simulink model "ctrl_custom"  (R2016b)
settings: Solver=ode4  StartTime=0.0  StopTime=inf  FixedStep=0.01  RelTol=1e-3  EnableMultiTasking=on
values from neighbouring files (symbols this model uses):
  T_pinv = T'*inv(T*T')    [initfile.m]
libraries: marine_gnc x8, simulink x1
(part 3 of 3)

== system ctrl_custom/Observer output /b_hat output ==
  b_hat : Inport
  Demux : Demux  Outputs=3
  b_psi_hat : S-Function  Priority=3  FunctionName=NIVeriStandIO  Parameters=width dtype portnum stime stype btype  SFunctionDeploymentMode=off  EnableBusSupport=off  mask(NI VeriStand Outport){portnum=3, width=-1, stime=-1, dtype=auto, stype=auto, btype=0}
      mask prompts: portnum "Port number:"; width "Port dimensions (-1 for dynamically sized):"; stime "Sample time (-1 for inherited):"; dtype "Data type:"; stype "Signal type:"; btype "Block type:"
      mask help: Use this outport on any level of nested subsystems to allow NI VeriStand software to map signals to it.
      mask init:
      | NIVeriStandIO_init;
      settings: CopyFcn=NIVeriStand_MDL_functions('', 'IO_copy');  DeleteFcn=NIVeriStand_MDL_functions('', 'IO_delete');  MoveFcn=set_param(gcb, 'Mask', 'on');
      mask Callback portnum: NIVeriStand_MDL_functions('', 'IO_setportnum');
      mask TypeOptions dtype: auto | double | single | int8 | uint8 | int16 | uint16 | int32 | uint32 | boolean
      mask Callback dtype: NIVeriStand_MDL_functions('', 'IO_booleansignal');
      mask TypeOptions stype: auto | real | complex
      mask Display:
      | patch([-x x], [-y y], [.90980 .81960 .32156]);
      | plot([xrad -x x xrad], [yrad -y y yrad]);
      | fprintf('NI Out%d', portnum);
  b_x_hat : S-Function  Priority=1  FunctionName=NIVeriStandIO  Parameters=width dtype portnum stime stype btype  SFunctionDeploymentMode=off  EnableBusSupport=off  mask(NI VeriStand Outport){portnum=1, width=-1, stime=-1, dtype=auto, stype=auto, btype=0}
      mask prompts: portnum "Port number:"; width "Port dimensions (-1 for dynamically sized):"; stime "Sample time (-1 for inherited):"; dtype "Data type:"; stype "Signal type:"; btype "Block type:"
      mask help: Use this outport on any level of nested subsystems to allow NI VeriStand software to map signals to it.
      mask init:
      | NIVeriStandIO_init;
      settings: CopyFcn=NIVeriStand_MDL_functions('', 'IO_copy');  DeleteFcn=NIVeriStand_MDL_functions('', 'IO_delete');  MoveFcn=set_param(gcb, 'Mask', 'on');
      mask Callback portnum: NIVeriStand_MDL_functions('', 'IO_setportnum');
      mask TypeOptions dtype: auto | double | single | int8 | uint8 | int16 | uint16 | int32 | uint32 | boolean
      mask Callback dtype: NIVeriStand_MDL_functions('', 'IO_booleansignal');
      mask TypeOptions stype: auto | real | complex
      mask Display:
      | patch([-x x], [-y y], [.90980 .81960 .32156]);
      | plot([xrad -x x xrad], [yrad -y y yrad]);
      | fprintf('NI Out%d', portnum);
  b_y_hat : S-Function  Priority=2  FunctionName=NIVeriStandIO  Parameters=width dtype portnum stime stype btype  SFunctionDeploymentMode=off  EnableBusSupport=off  mask(NI VeriStand Outport){portnum=2, width=-1, stime=-1, dtype=auto, stype=auto, btype=0}
      mask prompts: portnum "Port number:"; width "Port dimensions (-1 for dynamically sized):"; stime "Sample time (-1 for inherited):"; dtype "Data type:"; stype "Signal type:"; btype "Block type:"
      mask help: Use this outport on any level of nested subsystems to allow NI VeriStand software to map signals to it.
      mask init:
      | NIVeriStandIO_init;
      settings: CopyFcn=NIVeriStand_MDL_functions('', 'IO_copy');  DeleteFcn=NIVeriStand_MDL_functions('', 'IO_delete');  MoveFcn=set_param(gcb, 'Mask', 'on');
      mask Callback portnum: NIVeriStand_MDL_functions('', 'IO_setportnum');
      mask TypeOptions dtype: auto | double | single | int8 | uint8 | int16 | uint16 | int32 | uint32 | boolean
      mask Callback dtype: NIVeriStand_MDL_functions('', 'IO_booleansignal');
      mask TypeOptions stype: auto | real | complex
      mask Display:
      | patch([-x x], [-y y], [.90980 .81960 .32156]);
      | plot([xrad -x x xrad], [yrad -y y yrad]);
      | fprintf('NI Out%d', portnum);
  wires:
  Demux/1 -> b_x_hat/1
  Demux/2 -> b_y_hat/1
  Demux/3 -> b_psi_hat/1
  b_hat/1 -> Demux/1

== system ctrl_custom/Observer output /eta_hat output ==
  eta-_hat : Inport
  Demux : Demux  Outputs=3
  psi_hat : S-Function  Priority=3  FunctionName=NIVeriStandIO  Parameters=width dtype portnum stime stype btype  SFunctionDeploymentMode=off  EnableBusSupport=off  mask(NI VeriStand Outport){portnum=3, width=-1, stime=-1, dtype=auto, stype=auto, btype=0}
      mask prompts: portnum "Port number:"; width "Port dimensions (-1 for dynamically sized):"; stime "Sample time (-1 for inherited):"; dtype "Data type:"; stype "Signal type:"; btype "Block type:"
      mask help: Use this outport on any level of nested subsystems to allow NI VeriStand software to map signals to it.
      mask init:
      | NIVeriStandIO_init;
      settings: CopyFcn=NIVeriStand_MDL_functions('', 'IO_copy');  DeleteFcn=NIVeriStand_MDL_functions('', 'IO_delete');  MoveFcn=set_param(gcb, 'Mask', 'on');
      mask Callback portnum: NIVeriStand_MDL_functions('', 'IO_setportnum');
      mask TypeOptions dtype: auto | double | single | int8 | uint8 | int16 | uint16 | int32 | uint32 | boolean
      mask Callback dtype: NIVeriStand_MDL_functions('', 'IO_booleansignal');
      mask TypeOptions stype: auto | real | complex
      mask Display:
      | patch([-x x], [-y y], [.90980 .81960 .32156]);
      | plot([xrad -x x xrad], [yrad -y y yrad]);
      | fprintf('NI Out%d', portnum);
  x_hat : S-Function  Priority=1  FunctionName=NIVeriStandIO  Parameters=width dtype portnum stime stype btype  SFunctionDeploymentMode=off  EnableBusSupport=off  mask(NI VeriStand Outport){portnum=1, width=-1, stime=-1, dtype=auto, stype=auto, btype=0}
      mask prompts: portnum "Port number:"; width "Port dimensions (-1 for dynamically sized):"; stime "Sample time (-1 for inherited):"; dtype "Data type:"; stype "Signal type:"; btype "Block type:"
      mask help: Use this outport on any level of nested subsystems to allow NI VeriStand software to map signals to it.
      mask init:
      | NIVeriStandIO_init;
      settings: CopyFcn=NIVeriStand_MDL_functions('', 'IO_copy');  DeleteFcn=NIVeriStand_MDL_functions('', 'IO_delete');  MoveFcn=set_param(gcb, 'Mask', 'on');
      mask Callback portnum: NIVeriStand_MDL_functions('', 'IO_setportnum');
      mask TypeOptions dtype: auto | double | single | int8 | uint8 | int16 | uint16 | int32 | uint32 | boolean
      mask Callback dtype: NIVeriStand_MDL_functions('', 'IO_booleansignal');
      mask TypeOptions stype: auto | real | complex
      mask Display:
      | patch([-x x], [-y y], [.90980 .81960 .32156]);
      | plot([xrad -x x xrad], [yrad -y y yrad]);
      | fprintf('NI Out%d', portnum);
  y_hat : S-Function  Priority=2  FunctionName=NIVeriStandIO  Parameters=width dtype portnum stime stype btype  SFunctionDeploymentMode=off  EnableBusSupport=off  mask(NI VeriStand Outport){portnum=2, width=-1, stime=-1, dtype=auto, stype=auto, btype=0}
      mask prompts: portnum "Port number:"; width "Port dimensions (-1 for dynamically sized):"; stime "Sample time (-1 for inherited):"; dtype "Data type:"; stype "Signal type:"; btype "Block type:"
      mask help: Use this outport on any level of nested subsystems to allow NI VeriStand software to map signals to it.
      mask init:
      | NIVeriStandIO_init;
      settings: CopyFcn=NIVeriStand_MDL_functions('', 'IO_copy');  DeleteFcn=NIVeriStand_MDL_functions('', 'IO_delete');  MoveFcn=set_param(gcb, 'Mask', 'on');
      mask Callback portnum: NIVeriStand_MDL_functions('', 'IO_setportnum');
      mask TypeOptions dtype: auto | double | single | int8 | uint8 | int16 | uint16 | int32 | uint32 | boolean
      mask Callback dtype: NIVeriStand_MDL_functions('', 'IO_booleansignal');
      mask TypeOptions stype: auto | real | complex
      mask Display:
      | patch([-x x], [-y y], [.90980 .81960 .32156]);
      | plot([xrad -x x xrad], [yrad -y y yrad]);
      | fprintf('NI Out%d', portnum);
  wires:
  Demux/1 -> x_hat/1
  Demux/2 -> y_hat/1
  Demux/3 -> psi_hat/1
  eta-_hat/1 -> Demux/1

== system ctrl_custom/Observer output /nu_dot_hat output ==
  nu_dot_hat : Inport
  Demux : Demux  Outputs=3
  r_dot_hat : S-Function  Priority=3  FunctionName=NIVeriStandIO  Parameters=width dtype portnum stime stype btype  SFunctionDeploymentMode=off  EnableBusSupport=off  mask(NI VeriStand Outport){portnum=3, width=-1, stime=-1, dtype=auto, stype=auto, btype=0}
      mask prompts: portnum "Port number:"; width "Port dimensions (-1 for dynamically sized):"; stime "Sample time (-1 for inherited):"; dtype "Data type:"; stype "Signal type:"; btype "Block type:"
      mask help: Use this outport on any level of nested subsystems to allow NI VeriStand software to map signals to it.
      mask init:
      | NIVeriStandIO_init;
      settings: CopyFcn=NIVeriStand_MDL_functions('', 'IO_copy');  DeleteFcn=NIVeriStand_MDL_functions('', 'IO_delete');  MoveFcn=set_param(gcb, 'Mask', 'on');
      mask Callback portnum: NIVeriStand_MDL_functions('', 'IO_setportnum');
      mask TypeOptions dtype: auto | double | single | int8 | uint8 | int16 | uint16 | int32 | uint32 | boolean
      mask Callback dtype: NIVeriStand_MDL_functions('', 'IO_booleansignal');
      mask TypeOptions stype: auto | real | complex
      mask Display:
      | patch([-x x], [-y y], [.90980 .81960 .32156]);
      | plot([xrad -x x xrad], [yrad -y y yrad]);
      | fprintf('NI Out%d', portnum);
  u_dot_hat : S-Function  Priority=1  FunctionName=NIVeriStandIO  Parameters=width dtype portnum stime stype btype  SFunctionDeploymentMode=off  EnableBusSupport=off  mask(NI VeriStand Outport){portnum=1, width=-1, stime=-1, dtype=auto, stype=auto, btype=0}
      mask prompts: portnum "Port number:"; width "Port dimensions (-1 for dynamically sized):"; stime "Sample time (-1 for inherited):"; dtype "Data type:"; stype "Signal type:"; btype "Block type:"
      mask help: Use this outport on any level of nested subsystems to allow NI VeriStand software to map signals to it.
      mask init:
      | NIVeriStandIO_init;
      settings: CopyFcn=NIVeriStand_MDL_functions('', 'IO_copy');  DeleteFcn=NIVeriStand_MDL_functions('', 'IO_delete');  MoveFcn=set_param(gcb, 'Mask', 'on');
      mask Callback portnum: NIVeriStand_MDL_functions('', 'IO_setportnum');
      mask TypeOptions dtype: auto | double | single | int8 | uint8 | int16 | uint16 | int32 | uint32 | boolean
      mask Callback dtype: NIVeriStand_MDL_functions('', 'IO_booleansignal');
      mask TypeOptions stype: auto | real | complex
      mask Display:
      | patch([-x x], [-y y], [.90980 .81960 .32156]);
      | plot([xrad -x x xrad], [yrad -y y yrad]);
      | fprintf('NI Out%d', portnum);
  v_dot_hat : S-Function  Priority=2  FunctionName=NIVeriStandIO  Parameters=width dtype portnum stime stype btype  SFunctionDeploymentMode=off  EnableBusSupport=off  mask(NI VeriStand Outport){portnum=2, width=-1, stime=-1, dtype=auto, stype=auto, btype=0}
      mask prompts: portnum "Port number:"; width "Port dimensions (-1 for dynamically sized):"; stime "Sample time (-1 for inherited):"; dtype "Data type:"; stype "Signal type:"; btype "Block type:"
      mask help: Use this outport on any level of nested subsystems to allow NI VeriStand software to map signals to it.
      mask init:
      | NIVeriStandIO_init;
      settings: CopyFcn=NIVeriStand_MDL_functions('', 'IO_copy');  DeleteFcn=NIVeriStand_MDL_functions('', 'IO_delete');  MoveFcn=set_param(gcb, 'Mask', 'on');
      mask Callback portnum: NIVeriStand_MDL_functions('', 'IO_setportnum');
      mask TypeOptions dtype: auto | double | single | int8 | uint8 | int16 | uint16 | int32 | uint32 | boolean
      mask Callback dtype: NIVeriStand_MDL_functions('', 'IO_booleansignal');
      mask TypeOptions stype: auto | real | complex
      mask Display:
      | patch([-x x], [-y y], [.90980 .81960 .32156]);
      | plot([xrad -x x xrad], [yrad -y y yrad]);
      | fprintf('NI Out%d', portnum);
  wires:
  Demux/1 -> u_dot_hat/1
  Demux/2 -> v_dot_hat/1
  Demux/3 -> r_dot_hat/1
  nu_dot_hat/1 -> Demux/1

== system ctrl_custom/Observer output /nu_hat output ==
  nu_hat : Inport
  Demux : Demux  Outputs=3
  r_hat : S-Function  Priority=3  FunctionName=NIVeriStandIO  Parameters=width dtype portnum stime stype btype  SFunctionDeploymentMode=off  EnableBusSupport=off  mask(NI VeriStand Outport){portnum=3, width=-1, stime=-1, dtype=auto, stype=auto, btype=0}
      mask prompts: portnum "Port number:"; width "Port dimensions (-1 for dynamically sized):"; stime "Sample time (-1 for inherited):"; dtype "Data type:"; stype "Signal type:"; btype "Block type:"
      mask help: Use this outport on any level of nested subsystems to allow NI VeriStand software to map signals to it.
      mask init:
      | NIVeriStandIO_init;
      settings: CopyFcn=NIVeriStand_MDL_functions('', 'IO_copy');  DeleteFcn=NIVeriStand_MDL_functions('', 'IO_delete');  MoveFcn=set_param(gcb, 'Mask', 'on');
      mask Callback portnum: NIVeriStand_MDL_functions('', 'IO_setportnum');
      mask TypeOptions dtype: auto | double | single | int8 | uint8 | int16 | uint16 | int32 | uint32 | boolean
      mask Callback dtype: NIVeriStand_MDL_functions('', 'IO_booleansignal');
      mask TypeOptions stype: auto | real | complex
      mask Display:
      | patch([-x x], [-y y], [.90980 .81960 .32156]);
      | plot([xrad -x x xrad], [yrad -y y yrad]);
      | fprintf('NI Out%d', portnum);
  u_hat : S-Function  Priority=1  FunctionName=NIVeriStandIO  Parameters=width dtype portnum stime stype btype  SFunctionDeploymentMode=off  EnableBusSupport=off  mask(NI VeriStand Outport){portnum=1, width=-1, stime=-1, dtype=auto, stype=auto, btype=0}
      mask prompts: portnum "Port number:"; width "Port dimensions (-1 for dynamically sized):"; stime "Sample time (-1 for inherited):"; dtype "Data type:"; stype "Signal type:"; btype "Block type:"
      mask help: Use this outport on any level of nested subsystems to allow NI VeriStand software to map signals to it.
      mask init:
      | NIVeriStandIO_init;
      settings: CopyFcn=NIVeriStand_MDL_functions('', 'IO_copy');  DeleteFcn=NIVeriStand_MDL_functions('', 'IO_delete');  MoveFcn=set_param(gcb, 'Mask', 'on');
      mask Callback portnum: NIVeriStand_MDL_functions('', 'IO_setportnum');
      mask TypeOptions dtype: auto | double | single | int8 | uint8 | int16 | uint16 | int32 | uint32 | boolean
      mask Callback dtype: NIVeriStand_MDL_functions('', 'IO_booleansignal');
      mask TypeOptions stype: auto | real | complex
      mask Display:
      | patch([-x x], [-y y], [.90980 .81960 .32156]);
      | plot([xrad -x x xrad], [yrad -y y yrad]);
      | fprintf('NI Out%d', portnum);
  v_hat : S-Function  Priority=2  FunctionName=NIVeriStandIO  Parameters=width dtype portnum stime stype btype  SFunctionDeploymentMode=off  EnableBusSupport=off  mask(NI VeriStand Outport){portnum=2, width=-1, stime=-1, dtype=auto, stype=auto, btype=0}
      mask prompts: portnum "Port number:"; width "Port dimensions (-1 for dynamically sized):"; stime "Sample time (-1 for inherited):"; dtype "Data type:"; stype "Signal type:"; btype "Block type:"
      mask help: Use this outport on any level of nested subsystems to allow NI VeriStand software to map signals to it.
      mask init:
      | NIVeriStandIO_init;
      settings: CopyFcn=NIVeriStand_MDL_functions('', 'IO_copy');  DeleteFcn=NIVeriStand_MDL_functions('', 'IO_delete');  MoveFcn=set_param(gcb, 'Mask', 'on');
      mask Callback portnum: NIVeriStand_MDL_functions('', 'IO_setportnum');
      mask TypeOptions dtype: auto | double | single | int8 | uint8 | int16 | uint16 | int32 | uint32 | boolean
      mask Callback dtype: NIVeriStand_MDL_functions('', 'IO_booleansignal');
      mask TypeOptions stype: auto | real | complex
      mask Display:
      | patch([-x x], [-y y], [.90980 .81960 .32156]);
      | plot([xrad -x x xrad], [yrad -y y yrad]);
      | fprintf('NI Out%d', portnum);
  wires:
  Demux/1 -> u_hat/1
  Demux/2 -> v_hat/1
  Demux/3 -> r_hat/1
  nu_hat/1 -> Demux/1

== matlab function ctrl_custom/Projection [-pi,pi] to [-inf,inf] + shortest rotation/MATLAB Function11 ==
  data: alpha_prev input; alpha_infinf output; alpha_pipi input
function alpha_infinf  = fcn(alpha_prev,alpha_pipi)
alpha_infinf = NaN(6,1);

for i = 1:6
    % current rotation
    n = sign(alpha_prev(i)) * fix( (abs(alpha_prev(i))+pi)/(2*pi) ); 

    alpha_infinf(i) = 2*pi*n + alpha_pipi(i);

    alpha_tilde = alpha_infinf(i) - alpha_prev(i);

    % Shortest rotation
    if abs(alpha_tilde)>pi
        alpha_infinf(i) = alpha_infinf(i) - sign(alpha_tilde)*2*pi;
    end
end

end

== matlab function ctrl_custom/Input1/Control Gains/MATLAB Function ==
  data: u input; y output
function y = fcn(u)

y = diag(u);

== matlab function ctrl_custom/Thrust allocation: Pseudo-inverse of extended thrust configuration matrix/MATLAB Function11 ==
  data: u_e input; u output; alpha output
function [u, alpha]  = fcn(u_e)
u = [norm(u_e( 1: 2))
     norm(u_e( 3: 4))
     norm(u_e( 5: 6))
     norm(u_e( 7: 8))
     norm(u_e( 9:10))
     norm(u_e(11:12))];


alpha = [atan2(u_e( 2),u_e( 1))
         atan2(u_e( 4),u_e( 3))
         atan2(u_e( 6),u_e( 5))
         atan2(u_e( 8),u_e( 7))
         atan2(u_e(10),u_e( 9))
         atan2(u_e(12),u_e(11))];

end

== matlab function ctrl_custom/Input1/Control Gains/MATLAB Function1 ==
  data: u input; y output
function y = fcn(u)

y = diag(u);

== matlab function ctrl_custom/Input1/Control Gains/MATLAB Function2 ==
  data: u input; y output
function y = fcn(u)

y = diag(u);

== matlab function ctrl_custom/Input1/Guidance gains/MATLAB Function ==
  data: u input; y output
function y = fcn(u)

y = diag(u);

== matlab function ctrl_custom/Input1/Guidance gains/MATLAB Function1 ==
  data: u input; y output
function y = fcn(u)

y = diag(u);

== matlab function ctrl_custom/Input1/Observer Gains/MATLAB Function ==
  data: u input; y output
function y = fcn(u)

y = diag(u);

== matlab function ctrl_custom/Input1/Observer Gains/MATLAB Function1 ==
  data: u input; y output
function y = fcn(u)

y = diag(u);

== matlab function ctrl_custom/Input1/Observer Gains/MATLAB Function2 ==
  data: u input; y output
function y = fcn(u)

y = diag(u);

== matlab function ctrl_custom/Control/MATLAB Function ==
  data: K_p output; K_p1 input
function K_p = fcn(K_p1)
%#codegen

K_p = diag(K_p1);

== matlab function ctrl_custom/Control/MATLAB Function1 ==
  data: K_p output; K_p1 input
function K_p = fcn(K_p1)
%#codegen

K_p = diag(K_p1);

== matlab function ctrl_custom/Control/MATLAB Function4 ==
  data: Eta input; tau1 output; z_1 output; tau_L output; tau_U output; Chi_tilde output; nu input; Eta_t input; Eta_tdot input; Eta_tdotdot input; z_2 output; K_p input; K_d input
   function [ tau1,z_1,tau_L,tau_U,Chi_tilde,z_2] = Cascaded_feedback_controller_LP_LV(Eta,nu,Eta_t,Eta_tdot,Eta_tdotdot,K_p,K_d)
%  [ tau,theta ] = Adaptiv_controller(Eta,nu,nu_dot,phi,theta_t,Eta_d,Eta_dtheta,Eta_dtheta2,v_s,v_stheta,v_st,h)
%UNTITLED6 Summary of this function goes here Skjetne
%   Detailed explanation goes here
%kan være den må løses på en smartere måte
%include Model_c to path
%#codegen
persistent PHI OMEGA_N EPSI_RR EPSI_PHI RR PHIPHI p_r p_p S_old_RR S_old_PHI pp YY_r YY_phi


stored_data=20;
if (isempty(PHI)||isempty(OMEGA_N))
    PHI=zeros(8,1);
    OMEGA_N=zeros(3,1);
    PHIPHI=zeros(8,3*stored_data);
    RR=zeros(3,3*stored_data);
    EPSI_RR=zeros(3*stored_data,1);
    EPSI_PHI=zeros(3*stored_data,1);
    S_old_RR=0;
    S_old_PHI=0;
    p_r=1;
    p_p=1;
    pp=1;
    YY_r=zeros(3*stored_data,1);
    YY_phi=zeros(3*stored_data,1);
end

 m    = 127.92;%14.79;
 x_g  = 0;%0.0375;
 I_z  =  61.967;%1.7600;  
 
 X_ud  =    3.262; %-2.0;											% Table B.1
 Y_vd =     28.89;%-10.0;
 N_vd =    0.157;%-0.0;		% Table B.1
 Y_rd =    0.525;%  -0.0;
 N_rd =    13.98;%-1.0;		% Table B.1

    M_RB_c=[m     0      0;
          0     m      m*x_g;
          0     m*x_g  I_z];
    M_A_c=[-X_ud    0          0;
            0          -Y_vd  -Y_rd;
            0          -N_vd  -N_rd];     
    M_c=M_RB_c+M_A_c;
    
    %   
%% Damping coefficients
% Comments at the end of the lines indicate the old values used.
X_u		= -2.332;%-0.6555;		X_v		= 0;
X_uu 	= 0;%0.3545;		X_vv	= -2.443;
X_uuu 	= -8.557;%-3.787;		X_vvv	= 0;

						Y_v		= -4.673;%-1.33; 			Y_r		= -7.250; % Y_r
						Y_vv	= 0.3976;%-2.776;			Y_rr	= -3.450; % Y_rr
						Y_vvv	= 313.3;%-64.91;			Y_rrr	= 0;
				
                        Y_r		= 0;%-7.250; % Y_r
                        Y_rr	= 0;%-3.450; % Y_rr
                        Y_rrr	= 0;
                        
                        
						%Y_rv	= -0.805;			Y_vr	= -0.845; % Y_rv, Y_vr

						N_v		= 0;				%N_r		= -1.900; % N_r
						N_vv	= -0.2088;			%N_rr	= -0.750; % N_rr
						N_vvv	= 0;				%N_rrr	= 0;
						
                        N_r		= -0.01675;%-1.900; % N_r
                        N_rr	= -0.01148;%-0.750; % N_rr
                        N_rrr	= 0.0003578;%0;
						%N_rv	= 0.130;			N_vr	= 0.080; % N_rv, N_vr
    
    
    
R=Rot(Eta);

u   = nu(1);
v   = nu(2);
r   = nu(3);

d_11 = -X_u - X_uu*abs(u) - X_uuu*u^2;
d_22 = -Y_v - Y_vv*abs(v) - Y_vvv*v^2; %- Y_rv*abs(r);
d_33 = -N_r - N_rr*abs(r) - N_rrr*r^2; %- N_vr*abs(v); % using abs(r)

d_12 = 0;%-X_v - X_vv*v - X_vvv*v^2;
d_23 = -Y_r - Y_rr*abs(r) - Y_rrr*r^2;% - Y_vr*abs(v);
d_32 = -N_v - N_vv*abs(v) - N_vvv*v^2;% - N_rv*abs(r);

D    = [d_11 d_12 0
        0    d_22 d_23
        0    d_32 d_33];
  
%% controlsignaler
Eta_tilde=Eta-Eta_t;
Chi_tilde=Eta(3)-Eta_t(3);
Chi_tilde=mod(pi/2+Chi_tilde,pi)-pi/2; %%%%%%%%%%%%%%%%%%%%%%

%% New Controller
z_1=R'*(Eta_tilde);

Alpha_1=(-K_p*z_1+(R')*Eta_tdot);
z_2=nu-Alpha_1;

z_1_dot=S(nu)'*z_1-K_p*z_1+z_2;
Alpha_1dot=-K_p*z_1_dot+S(nu)'*R'*Eta_tdot + R'*Eta_tdotdot;

% TAU 
%tau=C_c(nu)*nu+D*nu+M_c*Alpha_1dot-K_d*z_2;
tau=M_c*Alpha_1dot-K_d*z_2;
tau1=tau;

%%
tau_L=-K_d*z_2+M_c*Alpha_1dot;
tau_U=C_c(nu)*nu+D*nu;

end

    function matrix=C_c(V) %%Coreolis matrix
    %#codegen
        matrix=C_RB_c(V)+C_A_c(V);
    end
      function matrix=C_RB_c(V)
      %#codegen
 m    = 127.92;%14.79;
 x_g  = 0;%0.0375;
 I_z  =  61.967;%1.7600;  
            u=V(1);
            v=V(2);
            r=V(3);
            matrix=[0        0       -m*(x_g*r+v);
                    0        0        m*u;
                    m*(x_g*r+v) -m*u    0]; 
      end
      function matrix=C_A_c(V)
      %#codegen
 X_ud  =    3.262; %-2.0;											% Table B.1
 Y_vd =     28.89;%-10.0;
 N_vd =    0.157;%-0.0;		% Table B.1
 Y_rd =    0.525;%  -0.0;
 N_rd =    13.98;%-1.0;		% Table B.1

            u=V(1);
            v=V(2);
            r=V(3);
        matrix=[0                                      0              Y_vd*v+0.5*(N_vd+Y_rd)*r;
               0                                       0             -X_ud*u;
               -Y_vd*v-0.5*(N_vd+Y_rd)*r         X_ud*u       0]; 
      end   
%{      
function [ d ] = G_d(nu)
      %#codegen
X_u		= -0.6555;
Y_v		= -1.33;
N_v		= 0;

    v=[nu(1) nu(2) 0]';

      D_L_uv=[-X_u    0  0 ;
            0     -Y_v 0;
            0     -N_v 0];
      d=(D_L_uv+D_NL_uv(v))*v;

end

function matrix = D_NL_uv(V)
      %#codegen


 
	
X_uu 	= 0.3545;		X_vv	= -2.443;
X_uuu 	= -3.787;	

			
Y_vv	= -2.776;			
Y_vvv	= -64.91;

N_vv	= -0.2088;	

    u=V(1);
    v=V(2);
    
     matrix=[-X_uu*abs(u)-X_uuu*u^2 0 0;
            0 -Y_vv*abs(v)-Y_vvv*v^2 0;
            0 -N_vv*abs(v) 0];
end
%}
function matrix=Rot(N)
      %#codegen

    yaw=N(3);
    matrix=[cos(yaw) -sin(yaw) 0;
            sin(yaw)  cos(yaw) 0;
            0         0        1]; 
end
%{
function R_d = Rot_dot(nu,eta)
%% takes in the nu vector 
      %#codegen


R_d=S([0 0 nu(3)])*Rot([0 0 eta(3)]);

end
%}
function [ s ] = S(r)
%UNTITLED2 Summary of this function goes here
%   Detailed explanation goes here
      %#codegen

s=[0 -r(3) r(2);
   r(3) 0 -r(1);
   -r(2) r(1) 0];

end
%{
function [ phi ] = Phi( nu )
%UNTITLED3 Summary of this function goes here
%   Detailed explanation goes here
      %#codegen

v=nu(2);
IvI=abs(v);
r=nu(3);
IrI=abs(r);

phi=[0 0 0 0 0 0 0 0;
     -IrI*v -r -IvI*r -IrI*r 0 0 0 0;
     0 0 0 0 -IrI*v -r -IvI*r -IrI*r];

end
%}

== matlab function ctrl_custom/Guidance/Reference model/w_d*w_d ==
  data: w_d input; y output
function y = fcn(w_d)
%#codegen

y = w_d*w_d;

== matlab function ctrl_custom/Guidance/Reference model/w_d*w_d1 ==
  data: w_d input; y output; zeta input
function y = fcn(w_d,zeta)
%#codegen

y = 2*zeta*w_d;

== matlab function ctrl_custom/Guidance/Reference model/w_d^-2 ==
  data: w_d input; y output
function y = fcn(w_d)
%#codegen

y = w_d^-2;

== matlab function ctrl_custom/Guidance/Reference model/w_d^3 ==
  data: w_d input; y output
function y = fcn(w_d)
%#codegen

y = w_d^3;

== matlab function ctrl_custom/Nonlinear Passisve Observer/C(nu)*nu ==
  data: nu_hat input; C_nl output
function C_nl = fcn(nu_hat)
%#codegen
u = nu_hat(1);
v = nu_hat(2);
r = nu_hat(3);

%% MATRICES
m    = 127.92;   x_g = 0; %0.0432;

%% Added mass
X_ud  =   3.262;	Y_vd =      28.89;		Y_rd =      0.525;

%% Correolis matrix
c_13 = -(m-Y_vd)*v-(m*x_g-Y_rd)*r;
c_23 = (m-X_ud)*u;

C    = [0     0     c_13
        0     0     c_23
        -c_13 -c_23 0   ];

    
C_NL = C;

C_nl =C_NL*nu_hat;

== matlab function ctrl_custom/Nonlinear Passisve Observer/D(nu)*nu ==
  data: nu_hat input; D_nl output
function D_nl = fcn(nu_hat)
%#codegen
u = nu_hat(1);
v = nu_hat(2);
r = nu_hat(3);

%% DAMPING 

% Surge:
% Based on fitting of towing data from -0.8 < u < 0.8 m/s
X_u     = -2.332;
X_uu	=  0;
X_uuu	= -8.557;

% Sway:
% Based on fitting of towing data from -0.45 < u < 0.45 m/s
Y_v 	= -4.673;
Y_vv	=  0.3976;
Y_vvv	= -313.3;

% Yaw:
% Based on fitting of towing data from -8 < u < 8 deg/s
% The fitting range is limited. Towing should be performed for higher
% velocities.
N_r		= -0.01675;
N_rr	= -0.01148;
N_rrr	= -0.0003578;

% Y_vvv og N_rrr er fra curvefitting uten minus, men ser ut til å fungere
% med minus. 
                           N_v		= 0;                Y_r	    =  -7.250; 
                           N_vv	    = -0.2088;          Y_rr	=  -3.450;
                           N_vvv	= 0;                Y_rrr	=  0;
						
						   Y_rv	    = -0.805;			Y_vr	=  -0.845; 

						   N_rv	    = 0.08;             N_vr	= 0.08;
                           
%% Assembly of the damping matrix
d_11 = X_u + X_uu*abs(u) + X_uuu*u^2;
d_22 = Y_v + Y_vv*abs(v) + Y_vvv*v^2;
d_33 = N_r + N_rr*abs(r) + N_rrr*r^2;

d_23 = 0; % Y_r + Y_rr*abs(r) + Y_rrr*r^2 + Y_vr*abs(v); Not verified, temporarily disabled
d_32 = 0; % N_v + N_vv*abs(v) + N_vvv*v^2 + N_rv*abs(r); Not verified, temporarily disabled

D    = - [d_11 0    0
          0    d_22 d_23
          0    d_32 d_33];


D_NL = D;

D_nl =D_NL*nu_hat;
